simulink model "roll_angle_holdautopilot"  (R2018b)
settings: Solver=VariableStepAuto  StartTime=0.0  StopTime=10  RelTol=1e-3
libraries: cstblocks x1
settings Model: Creator=FARYAL  LastModifiedBy=FARYAL

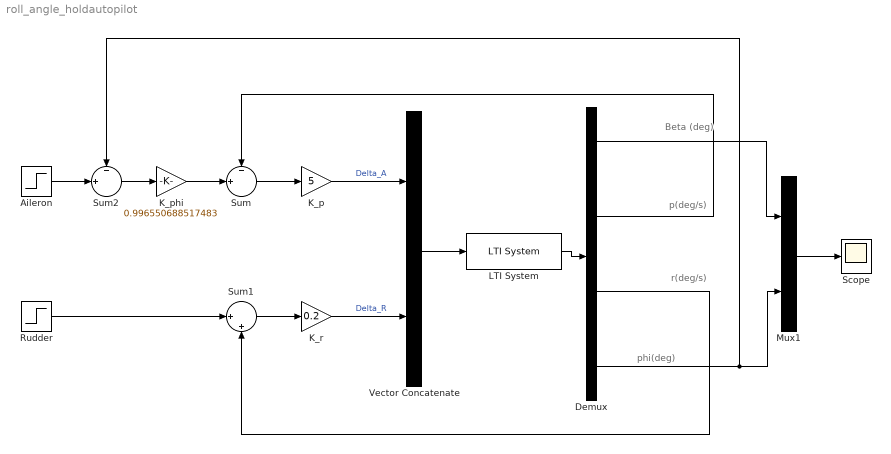
== system roll_angle_holdautopilot ==
  note: r(deg/s)
  note: phi(deg)
  note: p(deg/s)
  note: Beta (deg)
  "Aileron " : Step  SampleTime=0
  Demux : Demux
  K_p : Gain  Gain=5
  "K_phi " : Gain  Gain=0.996550688517483
  "K_r " : Gain  Gain=0.2
  LTI System : cstblocks/LTI System  sys=System  IC=[]
  Mux1 : Mux  Inputs=2
  "Rudder " : Step  After=0  SampleTime=0
  Scope : Scope
  Sum : Sum  Inputs=-|+||
  Sum1 : Sum  Inputs=||+|+
  Sum2 : Sum  Inputs=-|+||
  Vector Concatenate : Concatenate
  wires:
  LTI System/1 -> Demux/1
  Sum/1 -> K_p/1
  Vector Concatenate/1 -> LTI System/1
  Mux1/1 -> Scope/1
  K_p/1 -> Vector Concatenate/1  "Delta_A"
  Demux/1 -> Mux1/1
  Demux/2 -> Sum/1
  Sum1/1 -> "K_r "/1
  "K_r "/1 -> Vector Concatenate/2  "Delta_R"
  Demux/3 -> Sum1/2
  Demux/4 -> Mux1/2, Sum2/1
  Sum2/1 -> "K_phi "/1
  "Aileron "/1 -> Sum2/2
  "K_phi "/1 -> Sum/2
  "Rudder "/1 -> Sum1/1
